simulink model "SimulinkLab2Before"  (R2023b)
settings: Solver=VariableStepAuto  StartTime=0.0  StopTime=100  RelTol=1e-3
values from neighbouring files (symbols this model uses):
  Hf = tf(2,conv([1,1],[10,1]),'iodelay',1)    [IRA2Laborator2.m]
  Hpi_dis = c2d(Hpi,Te,'tustin')    [IRA2Laborator2.m]
  Hpi_dis_2 = c2d (Hpi, Te2, 'tustin')    [IRA2Laborator2.m]
settings Model: Creator=receaalex  LastModifiedBy=receaalex

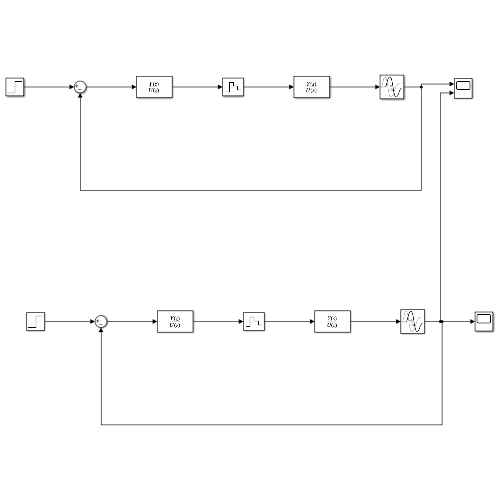
[thumbnail: Simulink's stored preview of the top-level diagram]
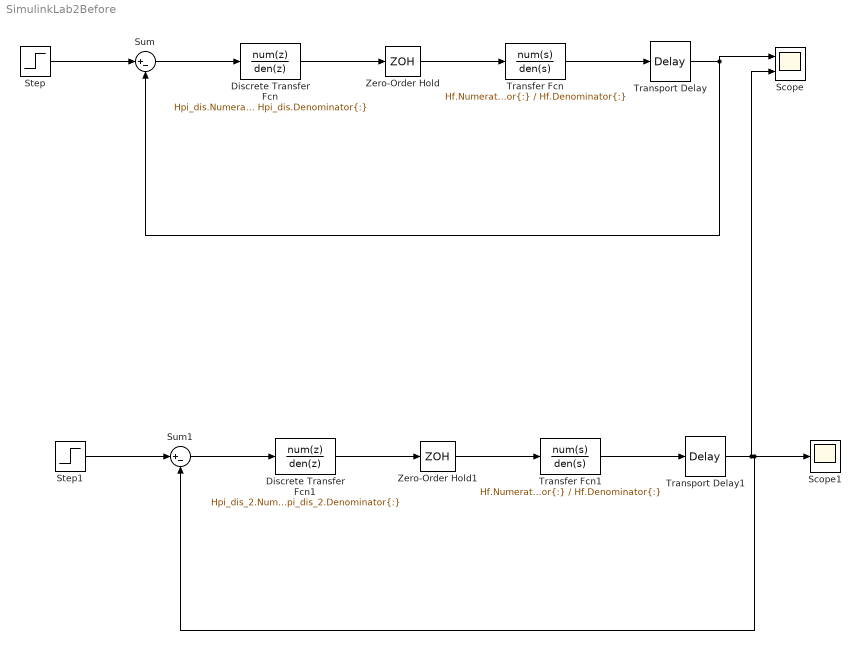
== system SimulinkLab2Before ==
  Discrete Transfer Fcn : DiscreteTransferFcn  Numerator=Hpi_dis.Numerator{:}  Denominator=Hpi_dis.Denominator{:}
  Discrete Transfer Fcn1 : DiscreteTransferFcn  Numerator=Hpi_dis_2.Numerator{:}  Denominator=Hpi_dis_2.Denominator{:}
  Scope : Scope  NumInputPorts=2
  Scope1 : Scope
  Step : Step  SampleTime=0
  Step1 : Step  SampleTime=0
  Sum : Sum  Inputs=|+-
  Sum1 : Sum  Inputs=|+-
  Transfer Fcn : TransferFcn  Numerator=Hf.Numerator{:}  Denominator=Hf.Denominator{:}
  Transfer Fcn1 : TransferFcn  Numerator=Hf.Numerator{:}  Denominator=Hf.Denominator{:}
  Transport Delay : TransportDelay
  Transport Delay1 : TransportDelay
  Zero-Order Hold : ZeroOrderHold  SampleTime=-1
  Zero-Order Hold1 : ZeroOrderHold  SampleTime=-1
  wires:
  Step/1 -> Sum/1
  Sum/1 -> Discrete Transfer Fcn/1
  Discrete Transfer Fcn/1 -> Zero-Order Hold/1
  Zero-Order Hold/1 -> Transfer Fcn/1
  Transfer Fcn/1 -> Transport Delay/1
  Transport Delay/1 -> Sum/2, Scope/1
  Transfer Fcn1/1 -> Transport Delay1/1
  Discrete Transfer Fcn1/1 -> Zero-Order Hold1/1
  Step1/1 -> Sum1/1
  Sum1/1 -> Discrete Transfer Fcn1/1
  Transport Delay1/1 -> Scope1/1, Sum1/2, Scope/2
  Zero-Order Hold1/1 -> Transfer Fcn1/1
